simulink model "model"  (R2023a)
settings: Solver=ode45  StartTime=0.0  StopTime=0.6  RelTol=1e-3  EnableMultiTasking=on
libraries: spsThreePhaseFaultLib x6, spsThreePhaseSourceLib x3, spsDistributedParametersLineLib x2, spsGroundLib x2, spsThreePhaseParallelRLCLoadLib x2, spsThreePhaseTransformer12TerminalsLib x2, spsThreePhaseSeriesRLCLoadLib x1, spsThreePhaseVIMeasurementLib x1, spspowerguiLib x1
settings Model: Creator=Administrator  LastModifiedBy=JOY
settings SolverCC: AlgebraicLoopSolver=TrustRegion
settings DataIOCC: LimitDataPoints=on  SaveFormat=Array  SignalLoggingSaveFormat=ModelDataLogs  ReturnWorkspaceOutputs=off
settings OptimizationCC: ExpressionDepthLimit=2147483647  LifeSpan=inf
settings DebuggingCC: UnderspecifiedInitializationDetection=Classic  MergeDetectMultiDrivingBlocksExec=none  SolverPrmCheckMsg=warning  FcnCallInpInsideContextMsg=warning  UnconnectedInputMsg=warning  UnconnectedOutputMsg=warning  UnconnectedLineMsg=warning  StateNameClashWarn=warning  SFUnexpectedBacktrackingDiag=warning  SFNoUnconditionalDefaultTransitionDiag=warning  SFExecutionAtInitializationDiag=none  ArithmeticOperatorsInVariantConditions=warning
settings HardwareCC: ProdBitPerPointer=32  ProdBitPerSizeT=32  ProdBitPerPtrDiffT=32  ProdLargestAtomicFloat=None  ProdIntDivRoundTo=Undefined  ProdEndianess=Unspecified  ProdWordSize=32  ProdHWDeviceType=32-bit Generic
settings ModelReferenceCC: EnableRefExpFcnMdlSchedulingChecks=on  PropagateSignalLabelsOutOfModel=off
settings SFSimCC: SimUseLocalCustomCode=off  CustomCodeUndefinedFunction=UseInterfaceOnly
settings RTWCC: RTWUseLocalCustomCode=off
settings CodeAppCC: StateflowObjectComments=on
settings GRTTargetCC: TargetLangStandard=C89/C90 (ANSI)  CombineOutputUpdateFcns=off  GRTInterface=on
settings ConfigComp: CovMetricSettings=dw  CovSaveCumulativeToWorkspaceVar=on  CovSaveSingleToWorkspaceVar=on  CovExternalEMLEnable=off  CovSFcnEnable=off
settings SimscapeCC: SimscapeNormalizeSystem=off

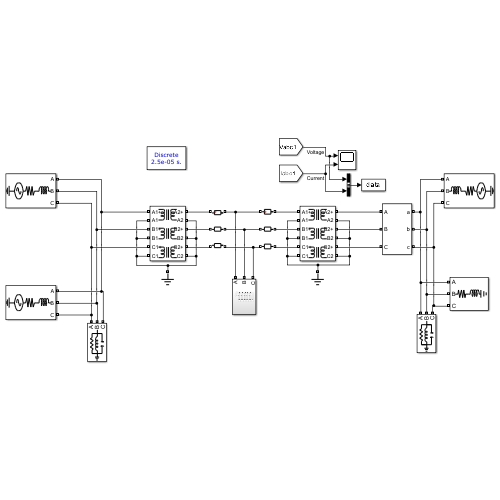
[thumbnail: Simulink's stored preview of the top-level diagram]
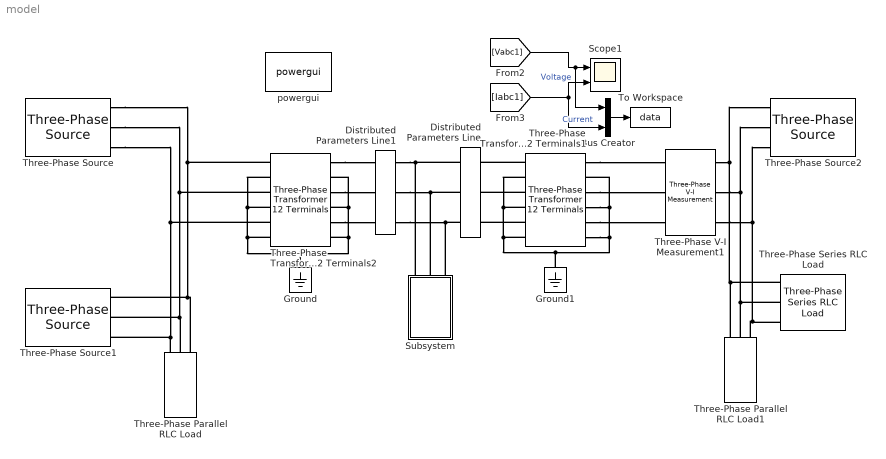
== system model ==
  Bus Creator : BusCreator  Inputs=2
  Distributed Parameters Line : spsDistributedParametersLineLib/Distributed Parameters Line  Phases=3  Length=33  Frequency=50  Resistance=[0.0132 0.132]  Inductance="[0.9337e-3  4.1264e-3]"  Capacitance=[12.74e-9 7.751e-9]  x1=[-0.0002 2.69003993742024e-10 0 0;-0.00015 2.65515011209444e-10 15635.7791244008 -78733.8101924461;-0.0001 2.61960516820835e-10 16870.5471169943 -78478.5008535488;-5e-05 2.58341387594499e-10 18101.1525545261 -78203.8281188648]  x2=[-0.0002 2.6391248407183e-10 0 0;-0.00015 2.59875167376894e-10 15586.3909292956 -78738.6897884679;-0.0001 2.55773730373004e-10 16821.2416601512 -78484.155603639;-5e-05 2.51609185028369e-10 18051.9420013289 -78210.2566277984]  x3=[-0.0002 6.14844150921262e-13 0 0;-0.00015 6.17215560963349e-13 51.7591743809053 -286.446961708194;-0.0001 6.19434682301364e-13 56.2521023005682 -285.598625681593;-5e-05 6.2150096740032e-13 60.7311508557067 -284.67982246761]  x4=[-0.0002 -2.67241963096722e-14 0 0;-0.00015 -2.71375397568363e-14 53.0400736803483 -296.594100248532;-0.0001 -2.75441874221332e-14 57.6922279035035 -295.72439290289;-5e-05 -2.79440389713362e-14 62.3301474326908 -294.781719988319]  x5=0.000186628717108595  V1=[2.547e-09 1.32e+05 1.32e+05;314.2 314.2 314.2;-0.1043 0.8095 -0.7613]  V2=[2.522e-09 1.32e+05 1.32e+05;314.2 314.2 314.2;-0.1193 0.8007 -0.7701]  I1=[2.615e-12 367.2 367.2;314.2 314.2 314.2;-0.5343 0.7771 -0.7937]  I2=[5.144e-12 607 607;314.2 314.2 314.2;-0.488 0.7934 -0.7774]  nHarmo=1  Measurements=None  Decoupling=off  VsMag0=0  VrMag0=0  VsAngle0=0  VrAngle0=0  IsMag0=0  IrMag0=0  IsAngle0=0  IrAngle0=0
      settings: LibrarySourceBlock=sps_lib/Power Grid Elements/Distributed Parameters Line
  Distributed Parameters Line1 : spsDistributedParametersLineLib/Distributed Parameters Line  Phases=3  Length=33  Frequency=50  Resistance=[0.0132 0.132]  Inductance="[0.9337e-3  4.1264e-3]"  Capacitance=[12.74e-9 7.751e-9]  x1=[-0.0002 2.89189780208285e-10 0 0;-0.00015 2.86119046498312e-10 15674.3204924212 -78626.6776409917;-0.0001 2.82977717194906e-10 16907.4009652816 -78370.7761372743;-5e-05 2.7976656737407e-10 18136.3097899448 -78095.5378172321]  x2=[-0.0002 2.69118209031691e-10 0 0;-0.00015 2.65600697344123e-10 15635.7791244008 -78733.8101924461;-0.0001 2.62017652658755e-10 16870.5471169943 -78478.5008535488;-5e-05 2.58369959038248e-10 18101.1525545261 -78203.8281188648]  x3=[-0.0002 8.3031268797308e-13 0 0;-0.00015 8.14306603244767e-13 41.4228708035809 -287.645866206953;-0.0001 7.98099600546835e-13 45.9359054607536 -286.959737874601;-5e-05 7.81695678714688e-13 50.4376061206075 -286.202806520798]  x4=[-0.0002 2.76583260192225e-13 0 0;-0.00015 2.78383387858809e-13 63.708177517744 -294.987739785216;-0.0001 2.80114828589978e-13 68.3337840298888 -293.950663320189;-5e-05 2.81777155178641e-13 72.9425302033246 -292.841058927466]  x5=0.000186628717108595  V1=[2.618e-09 1.319e+05 1.319e+05;314.2 314.2 314.2;-0.1003 0.8184 -0.7524]  V2=[2.549e-09 1.32e+05 1.32e+05;314.2 314.2 314.2;-0.1043 0.8095 -0.7613]  I1=[2.387e-12 367.3 367.3;314.2 314.2 314.2;0.1434 0.7414 -0.8294]  I2=[6.175e-12 607.4 607.4;314.2 314.2 314.2;-0.4569 0.8292 -0.7416]  nHarmo=1  Measurements=None  Decoupling=off  VsMag0=0  VrMag0=0  VsAngle0=0  VrAngle0=0  IsMag0=0  IrMag0=0  IsAngle0=0  IrAngle0=0
      settings: LibrarySourceBlock=sps_lib/Power Grid Elements/Distributed Parameters Line
  Ground : spsGroundLib/Ground  LConnTagsString=a
  Ground1 : spsGroundLib/Ground  LConnTagsString=a
  Scope1 : Scope  NumInputPorts=2
  Subsystem : Subsystem
  Three-Phase Parallel RLC Load : spsThreePhaseParallelRLCLoadLib/Three-Phase Parallel RLC Load  LConnTagsString=A|B|C  Configuration=Y (grounded)  NominalVoltage=1000  Vabc=[1e3 1e3 1e3]  Vabcp=[1e3 1e3 1e3]  NominalFrequency=60  UnbalancedPower=off  ActivePower=10e4  InductivePower=100  CapacitivePower=100  Pabc=[10e3 9e3 11e3]  QLabc=[100 90 110]  QCabc=[100 90 110]  Pabcp=[10e3 9e3 11e3]  QLabcp=[100 90 110]  QCabcp=[100 90 110]  Measurements=None  LoadType=constant Z
  Three-Phase Parallel RLC Load1 : spsThreePhaseParallelRLCLoadLib/Three-Phase Parallel RLC Load  LConnTagsString=A|B|C  Configuration=Y (grounded)  NominalVoltage=1000  Vabc=[1e3 1e3 1e3]  Vabcp=[1e3 1e3 1e3]  NominalFrequency=60  UnbalancedPower=off  ActivePower=100  InductivePower=10  CapacitivePower=10  Pabc=[10e3 9e3 11e3]  QLabc=[100 90 110]  QCabc=[100 90 110]  Pabcp=[10e3 9e3 11e3]  QLabcp=[100 90 110]  QCabcp=[100 90 110]  Measurements=None  LoadType=constant Z
  Three-Phase Series RLC Load : spsThreePhaseSeriesRLCLoadLib/Three-Phase Series RLC Load  LConnTagsString=A|B|C  Configuration=Y (grounded)  NominalVoltage=11e3  Vabc=[1e3 1e3 1e3]  Vabcp=[1e3 1e3 1e3]  NominalFrequency=50  UnbalancedPower=off  ActivePower=10e6  InductivePower=100  CapacitivePower=0  Pabc=[10e3 9e3 11e3]  QLabc=[100 90 110]  QCabc=[100 90 110]  Pabcp=[10e3 9e3 11e3]  QLabcp=[100 90 110]  QCabcp=[100 90 110]  Measurements=None  LoadType=constant Z
  Three-Phase V-I Measurement1 : spsThreePhaseVIMeasurementLib/Three-Phase V-I Measurement  VoltageMeasurement=phase-to-phase  SetLabelV=on  LabelV=Vabc1  Vpu=off  VpuLL=on  CurrentMeasurement=yes  SetLabelI=on  LabelI=Iabc1  Ipu=off  Pbase=100e6  Vbase=11e3  OutputType=Complex  PhasorSimulation=off  PSBequivalent=0
  Three-Phase Source : spsThreePhaseSourceLib/Three-Phase Source  InternalConnection=Yg  VoltagePhases=off  Voltage=11e3  PhaseAngle=0  Voltage_phases=[25e3 25e3 25e3]/sqrt(3)  PhaseAngles_phases=[0 -120 +120]  Frequency=50  NonIdealSource=on  SpecifyImpedance=off  Resistance=12  Inductance=16.58e-3  ShortCircuitLevel=50e6  BaseVoltage=11e3  XRratio=7  BusType=PV  Pref=50e6  Qref=0  Prefabc=[10e3, 10e3, 10e3]  Qrefabc=[0, 0, 0]  Qmin=-inf  Qmax=inf
  Three-Phase Source1 : spsThreePhaseSourceLib/Three-Phase Source  InternalConnection=Yg  VoltagePhases=off  Voltage=11e3  PhaseAngle=0  Voltage_phases=[25e3 25e3 25e3]/sqrt(3)  PhaseAngles_phases=[0 -120 +120]  Frequency=50  NonIdealSource=on  SpecifyImpedance=off  Resistance=12  Inductance=16.58e-3  ShortCircuitLevel=50e6  BaseVoltage=11e3  XRratio=7  BusType=PV  Pref=50e6  Qref=0  Prefabc=[10e3, 10e3, 10e3]  Qrefabc=[0, 0, 0]  Qmin=-inf  Qmax=inf
  Three-Phase Source2 : spsThreePhaseSourceLib/Three-Phase Source  InternalConnection=Yg  VoltagePhases=off  Voltage=11e3  PhaseAngle=0  Voltage_phases=[25e3 25e3 25e3]/sqrt(3)  PhaseAngles_phases=[0 -120 +120]  Frequency=50  NonIdealSource=on  SpecifyImpedance=off  Resistance=8.4  Inductance=16.58e-3  ShortCircuitLevel=20e6  BaseVoltage=11e3  XRratio=7  BusType=PV  Pref=20e6  Qref=0  Prefabc=[10e3, 10e3, 10e3]  Qrefabc=[0, 0, 0]  Qmin=-inf  Qmax=inf
  Three-Phase Transformer 12 Terminals1 : spsThreePhaseTransformer12TerminalsLib/Three-Phase Transformer 12 Terminals  RatedPower=[100e6 50]  Winding1="[ 132e3 0.002  0.05 ]"  Winding2=[ 11e3 0.002 0.05]  RmXm=[ 200 200 ]
      settings: LibrarySourceBlock=|
      | sps_lib/Power Grid Elements/Three-Phase Transformer
      | 12 Terminals
  Three-Phase Transformer 12 Terminals2 : spsThreePhaseTransformer12TerminalsLib/Three-Phase Transformer 12 Terminals  RatedPower=[100e6 50]  Winding1="[ 11e3 0.002  0.05 ]"  Winding2=[ 132e3 0.002 0.05]  RmXm=[ 200 200 ]
      settings: LibrarySourceBlock=|
      | sps_lib/Power Grid Elements/Three-Phase Transformer
      | 12 Terminals
  To Workspace : ToWorkspace  VariableName=data  SaveFormat=Structure With Time  SampleTime=-1
  powergui : spspowerguiLib/powergui  Priority=1  SimulationMode=Discrete  SampleTime=25e-6  frequency=60  Iterations=50  frequencyindice=50  Pbase=100e6  ErrMax=1e-4  UnitsV=kV  UnitsW=MW  buscounter=0  FunctionMessages=off  echomessages=off  EnableUseOfTLC=off  CurrentSourceSwitches=off  DisableSnubberDevices=off  DisableRonSwitches=off  DisableVfSwitches=off  DisplayEquations=off  AutomaticDiscreteSolvers=off  SolverType=Tustin  Interpol=off  ExternalGateDelay=off  methode=off  Ts=0  x0status=blocks  SPID=off  SwTol=0  HookPort=off  NonlinearTolerance=1e-4  nMaxIteration=100  ContinueOnMaxIteration=off  RestoreLinks=warning  ResistiveCurrentMeasurement=off  Frange=[0:2:500]  Ylog=off  Xlog=on  ShowGrid=off  save=off  variable=ZData  structure=0  ZoomFFT=off  StartTime=0.0  cycles=1  DisplayStyle=1  fundamental=60  FreqAxis=off  MaxFrequency=1000  frequencyindicesteady=1  RmsSteady=1  display=off
  wires:
  [Vabc1] -> Bus Creator/1, Scope1/1  "Voltage"
  [Iabc1] -> Bus Creator/2, Scope1/2  "Current"
  Bus Creator/1 -> To Workspace/1
  connections:
  Distributed Parameters Line/LConn1 -- Distributed Parameters Line1/RConn1 -- Subsystem/LConn1
  Three-Phase Series RLC Load/LConn2 -- Three-Phase Parallel RLC Load1/LConn2 -- Three-Phase V-I Measurement1/RConn2 -- Three-Phase Source2/RConn2
  Distributed Parameters Line/LConn3 -- Distributed Parameters Line1/RConn3 -- Subsystem/LConn3
  Three-Phase Series RLC Load/LConn1 -- Three-Phase Parallel RLC Load1/LConn1 -- Three-Phase V-I Measurement1/RConn1 -- Three-Phase Source2/RConn1
  Distributed Parameters Line/LConn2 -- Subsystem/LConn2 -- Distributed Parameters Line1/RConn2
  Three-Phase Series RLC Load/LConn3 -- Three-Phase Parallel RLC Load1/LConn3 -- Three-Phase V-I Measurement1/RConn3 -- Three-Phase Source2/RConn3
  Three-Phase Transformer 12 Terminals1/LConn3 -- Distributed Parameters Line/RConn2
  Three-Phase Transformer 12 Terminals1/LConn1 -- Distributed Parameters Line/RConn1
  Three-Phase Transformer 12 Terminals1/LConn5 -- Distributed Parameters Line/RConn3
  Three-Phase Transformer 12 Terminals2/RConn1 -- Distributed Parameters Line1/LConn1
  Three-Phase Transformer 12 Terminals2/RConn3 -- Distributed Parameters Line1/LConn2
  Three-Phase Transformer 12 Terminals2/RConn5 -- Distributed Parameters Line1/LConn3
  Three-Phase Source/RConn2 -- Three-Phase Parallel RLC Load/LConn2 -- Three-Phase Source1/RConn2 -- Three-Phase Transformer 12 Terminals2/LConn3
  Three-Phase Source/RConn1 -- Three-Phase Parallel RLC Load/LConn3 -- Three-Phase Source1/RConn1 -- Three-Phase Transformer 12 Terminals2/LConn1
  Three-Phase Source/RConn3 -- Three-Phase Parallel RLC Load/LConn1 -- Three-Phase Source1/RConn3 -- Three-Phase Transformer 12 Terminals2/LConn5
  Three-Phase Transformer 12 Terminals1/RConn5 -- Three-Phase V-I Measurement1/LConn3
  Three-Phase Transformer 12 Terminals1/RConn3 -- Three-Phase V-I Measurement1/LConn2
  Three-Phase Transformer 12 Terminals1/RConn1 -- Three-Phase V-I Measurement1/LConn1
  Ground/LConn1 -- Three-Phase Transformer 12 Terminals2/LConn6 -- Three-Phase Transformer 12 Terminals2/LConn4 -- Three-Phase Transformer 12 Terminals2/LConn2 -- Three-Phase Transformer 12 Terminals2/RConn6 -- Three-Phase Transformer 12 Terminals2/RConn4 -- Three-Phase Transformer 12 Terminals2/RConn2
  Ground1/LConn1 -- Three-Phase Transformer 12 Terminals1/LConn2 -- Three-Phase Transformer 12 Terminals1/LConn4 -- Three-Phase Transformer 12 Terminals1/LConn6 -- Three-Phase Transformer 12 Terminals1/RConn6 -- Three-Phase Transformer 12 Terminals1/RConn4 -- Three-Phase Transformer 12 Terminals1/RConn2

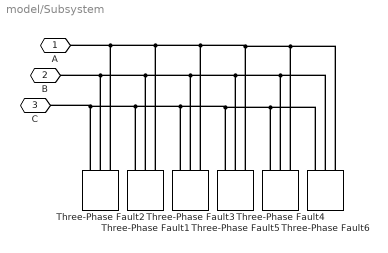
== system model/Subsystem ==
  Three-Phase Fault1 : spsThreePhaseFaultLib/Three-Phase Fault  InitialStates=0  FaultA=on  FaultB=on  FaultC=off  GroundFault=on  SwitchTimes=[ 0.125 0.175]  External=off  SwitchStatus=NaN  FaultResistance=0.001  GroundResistance=0.001  SnubberResistance=1e6  SnubberCapacitance=inf  Measurements=None
  Three-Phase Fault2 : spsThreePhaseFaultLib/Three-Phase Fault  InitialStates=0  FaultA=on  FaultB=off  FaultC=off  GroundFault=on  SwitchTimes=[ 0.025 0.075]  External=off  SwitchStatus=NaN  FaultResistance=0.001  GroundResistance=0.001  SnubberResistance=1e6  SnubberCapacitance=inf  Measurements=None
  Three-Phase Fault3 : spsThreePhaseFaultLib/Three-Phase Fault  InitialStates=0  FaultA=off  FaultB=on  FaultC=on  GroundFault=off  SwitchTimes=[ 0.225 0.275]  External=off  SwitchStatus=NaN  FaultResistance=0.001  GroundResistance=0.001  SnubberResistance=1e6  SnubberCapacitance=inf  Measurements=None
  Three-Phase Fault4 : spsThreePhaseFaultLib/Three-Phase Fault  InitialStates=0  FaultA=on  FaultB=on  FaultC=on  GroundFault=on  SwitchTimes=[ 0.425 0.475]  External=off  SwitchStatus=NaN  FaultResistance=0.001  GroundResistance=0.001  SnubberResistance=1e6  SnubberCapacitance=inf  Measurements=None
  Three-Phase Fault5 : spsThreePhaseFaultLib/Three-Phase Fault  InitialStates=0  FaultA=on  FaultB=on  FaultC=on  GroundFault=off  SwitchTimes=[ 0.325 0.375]  External=off  SwitchStatus=NaN  FaultResistance=0.001  GroundResistance=0.001  SnubberResistance=1e6  SnubberCapacitance=inf  Measurements=None
  Three-Phase Fault6 : spsThreePhaseFaultLib/Three-Phase Fault  InitialStates=0  FaultA=off  FaultB=off  FaultC=off  GroundFault=off  SwitchTimes=[ 0.525 0.575]  External=off  SwitchStatus=NaN  FaultResistance=0.001  GroundResistance=0.001  SnubberResistance=1e6  SnubberCapacitance=inf  Measurements=None
  A : PMIOPort  Side=Left
  B : PMIOPort  Port=2  Side=Left
  C : PMIOPort  Port=3  Side=Left
  connections:
  Three-Phase Fault2/LConn2 -- Three-Phase Fault6/LConn2 -- Three-Phase Fault4/LConn2 -- Three-Phase Fault5/LConn2 -- Three-Phase Fault3/LConn2 -- Three-Phase Fault1/LConn2 -- B/RConn1
  Three-Phase Fault2/LConn3 -- Three-Phase Fault6/LConn3 -- Three-Phase Fault4/LConn3 -- Three-Phase Fault5/LConn3 -- Three-Phase Fault3/LConn3 -- Three-Phase Fault1/LConn3 -- C/RConn1
  Three-Phase Fault2/LConn1 -- Three-Phase Fault6/LConn1 -- Three-Phase Fault4/LConn1 -- Three-Phase Fault5/LConn1 -- Three-Phase Fault3/LConn1 -- Three-Phase Fault1/LConn1 -- A/RConn1
